simulink library "mechLibrary"  (R2019a)
settings: Solver=VariableStepAuto  StartTime=0.0  StopTime=10.0  RelTol=1e-3
undefined symbols (not defined in the file): X, Y, Z
libraries: sm_lib x45, fl_lib x16, nesl_utility x14, $bdroot x8, servoLibrary x6
(part 1 of 2)
Description:
  | Copyright 2008-2019 The MathWorks, Inc.
  | 
  | Mechanical library
settings Model: Creator=falderis  LastModifiedBy=falderis
settings DataIOCC: ReturnWorkspaceOutputs=off
settings DebuggingCC: ArithmeticOperatorsInVariantConditions=warning

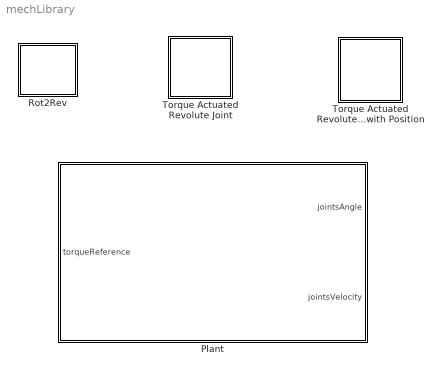
== system mechLibrary ==
  Plant : Subsystem  Description=|
      | Copyright 2008-2019 The MathWorks, Inc.
      | 
      | Mechanical library
      mask Display: image('plant.png')
  Rot2Rev : Subsystem
  Torque Actuated Revolute Joint : Subsystem  mask(Torque actuated revolute joint){angle=0}
      mask prompts: angle "State target for revolute joint (deg)"
      mask Display: image('rev.png');
  Torque Actuated Revolute Joint with Position : Subsystem  mask(Torque actuated revolute joint){angle=0}
      mask prompts: angle "State target for revolute joint (deg)"
      mask Display: image('rev.png');

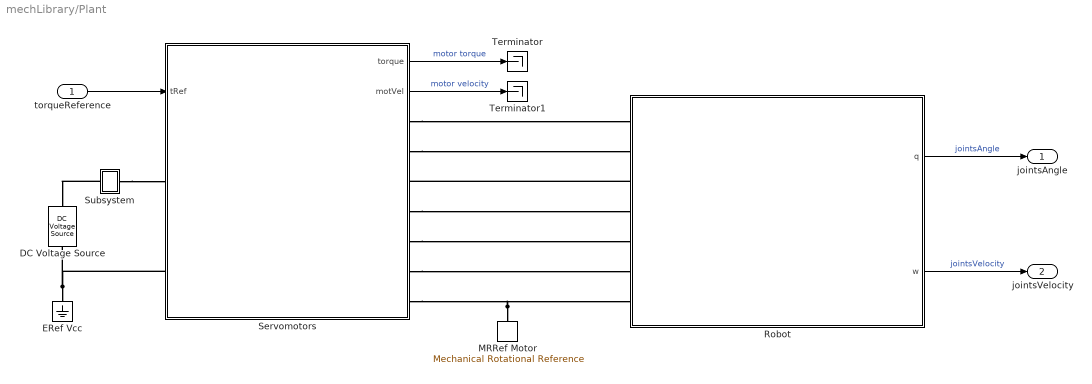
== system mechLibrary/Plant ==
  torqueReference : Inport  OutDataTypeStr=Bus: jointTorqueBus  Unit=N*m
  DC Voltage Source : fl_lib/Electrical/Electrical Sources/DC Voltage Source  v0=12 V
  ERef Vcc : fl_lib/Electrical/Electrical Elements/Electrical Reference
      settings: SourceProductName=Foundation Library
  MRRef Motor : fl_lib/Mechanical/Rotational Elements/Mechanical Rotational Reference
      settings: SourceProductName=Foundation Library
  Robot : Subsystem
      mask Display: image(imread(fullfile(matlabroot,'toolbox','physmod','sm','smdemos','import','robot_stepfiles','images','sm_srobot.png')))
  Servomotors : Subsystem  VariantControl=SV
      mask Display: image('servos.jpg')
  Subsystem : Subsystem
      mask Display: disp('i')
  Terminator : Terminator
  Terminator1 : Terminator
  jointsAngle : Outport  OutDataTypeStr=Bus: jointMotionBus  Unit=deg
  jointsVelocity : Outport  Port=2  OutDataTypeStr=Bus: jointVelBus  Unit=deg/s
  wires:
  Robot/2(w) -> jointsVelocity/1  "jointsVelocity"
  Robot/1(q) -> jointsAngle/1  "jointsAngle"
  Servomotors/2(motVel) -> Terminator1/1  "motor velocity"
  torqueReference/1 -> Servomotors/1(tRef)
  Servomotors/1(torque) -> Terminator/1  "motor torque"
  connections:
  Subsystem/LConn1 -- DC Voltage Source/LConn1
  Subsystem/RConn1 -- Servomotors/LConn1
  Servomotors/RConn6 -- Robot/LConn6
  Servomotors/RConn5 -- Robot/LConn5
  Servomotors/RConn4 -- Robot/LConn4
  Robot/LConn3 -- Servomotors/RConn3
  Servomotors/RConn2 -- Robot/LConn2
  Servomotors/RConn1 -- Robot/LConn1
  ERef Vcc/LConn1 -- DC Voltage Source/RConn1 -- Servomotors/LConn2
  MRRef Motor/LConn1 -- Robot/LConn7 -- Servomotors/RConn7

== system mechLibrary/Rot2Rev ==
  Ideal Angular Velocity Source : fl_lib/Mechanical/Mechanical Sources/Ideal Angular Velocity Source
  Ideal Torque Sensor : fl_lib/Mechanical/Mechanical Sensors/Ideal Torque Sensor
  w : PMIOPort  Side=Right
  R : PMIOPort  Port=2  Side=Right
  t : PMIOPort  Port=3  Side=Left
  C : PMIOPort  Port=4  Side=Left
  connections:
  Ideal Torque Sensor/LConn1 -- Ideal Angular Velocity Source/RConn2
  Ideal Torque Sensor/RConn2 -- t/RConn1
  C/RConn1 -- Ideal Torque Sensor/RConn1
  w/RConn1 -- Ideal Angular Velocity Source/RConn1
  Ideal Angular Velocity Source/LConn1 -- R/RConn1

== system mechLibrary/Torque Actuated Revolute Joint ==
  Rot2Rev : $bdroot/Rot2Rev  SystemSampleTime=-1
  Upper Arm Revolute : sm_lib/Joints/Revolute Joint  SenseConstraintForce=off  SenseConstraintForceX=off  SenseConstraintForceY=off  SenseConstraintForceZ=off  SenseConstraintTorque=off  SenseConstraintTorqueX=off  SenseConstraintTorqueY=off  SenseConstraintTorqueZ=off  SenseTotalForce=off  SenseTotalForceX=off  SenseTotalForceY=off  SenseTotalForceZ=off  SenseTotalTorque=off  SenseTotalTorqueX=off  SenseTotalTorqueY=off  SenseTotalTorqueZ=off  CompositeWrenchDir=FollowerOnBase  CompositeWrenchFrame=BaseFrame  EquilibriumPosition=0  EquilibriumPositionUnits=deg  SpringStiffness=0  SpringStiffnessUnits=N*m/deg  DampingCoefficient=0  DampingCoefficientUnits=N*m/(deg/s)  TorqueActuationMode=InputTorque  MotionActuationMode=ComputedMotion  SensePosition=off  SenseVelocity=on  SenseAcceleration=off  SenseTorqueForce=off  SenseLowerLimitTorqueForce=off  SenseUpperLimitTorqueForce=off  LowerLimitSpecify=off  LowerLimitBound=-90  LowerLimitBoundUnits=deg  LowerLimitStiffness=1e4  LowerLimitStiffnessUnits=N*m/deg  LowerLimitDamping=10  LowerLimitDampingUnits=N*m/(deg/s)  LowerLimitTransitionRegionWidth=0.1  LowerLimitTransitionRegionWidthUnits=deg  UpperLimitSpecify=off  UpperLimitBound=90  UpperLimitBoundUnits=deg  UpperLimitStiffness=1e4  UpperLimitStiffnessUnits=N*m/deg  UpperLimitDamping=10  UpperLimitDampingUnits=N*m/(deg/s)  UpperLimitTransitionRegionWidth=0.1  UpperLimitTransitionRegionWidthUnits=deg  PositionTargetSpecify=on  PositionTargetPriority=Low  PositionTargetValue=angle  PositionTargetValueUnits=deg  VelocityTargetSpecify=off  VelocityTargetPriority=High  VelocityTargetValue=0  VelocityTargetValueUnits=deg/s
  F : PMIOPort  Side=Right
  B : PMIOPort  Port=2  Side=Left
  C : PMIOPort  Port=3  Side=Left
  w : PMIOPort  Port=4  Side=Right
  R : PMIOPort  Port=5  Side=Right
  connections:
  Upper Arm Revolute/RConn2 -- w/RConn1 -- Rot2Rev/RConn1
  Rot2Rev/RConn2 -- R/RConn1
  F/RConn1 -- Upper Arm Revolute/RConn1
  Rot2Rev/LConn1 -- Upper Arm Revolute/LConn2
  B/RConn1 -- Upper Arm Revolute/LConn1
  Rot2Rev/LConn2 -- C/RConn1

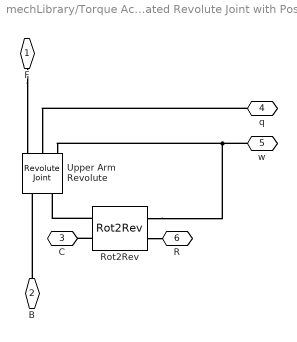
== system mechLibrary/Torque Actuated Revolute Joint with Position ==
  Rot2Rev : $bdroot/Rot2Rev  SystemSampleTime=-1
  Upper Arm Revolute : sm_lib/Joints/Revolute Joint  SenseConstraintForce=off  SenseConstraintForceX=off  SenseConstraintForceY=off  SenseConstraintForceZ=off  SenseConstraintTorque=off  SenseConstraintTorqueX=off  SenseConstraintTorqueY=off  SenseConstraintTorqueZ=off  SenseTotalForce=off  SenseTotalForceX=off  SenseTotalForceY=off  SenseTotalForceZ=off  SenseTotalTorque=off  SenseTotalTorqueX=off  SenseTotalTorqueY=off  SenseTotalTorqueZ=off  CompositeWrenchDir=FollowerOnBase  CompositeWrenchFrame=BaseFrame  EquilibriumPosition=0  EquilibriumPositionUnits=deg  SpringStiffness=0  SpringStiffnessUnits=N*m/deg  DampingCoefficient=0  DampingCoefficientUnits=N*m/(deg/s)  TorqueActuationMode=InputTorque  MotionActuationMode=ComputedMotion  SensePosition=on  SenseVelocity=on  SenseAcceleration=off  SenseTorqueForce=off  SenseLowerLimitTorqueForce=off  SenseUpperLimitTorqueForce=off  LowerLimitSpecify=off  LowerLimitBound=-90  LowerLimitBoundUnits=deg  LowerLimitStiffness=1e4  LowerLimitStiffnessUnits=N*m/deg  LowerLimitDamping=10  LowerLimitDampingUnits=N*m/(deg/s)  LowerLimitTransitionRegionWidth=0.1  LowerLimitTransitionRegionWidthUnits=deg  UpperLimitSpecify=off  UpperLimitBound=90  UpperLimitBoundUnits=deg  UpperLimitStiffness=1e4  UpperLimitStiffnessUnits=N*m/deg  UpperLimitDamping=10  UpperLimitDampingUnits=N*m/(deg/s)  UpperLimitTransitionRegionWidth=0.1  UpperLimitTransitionRegionWidthUnits=deg  PositionTargetSpecify=on  PositionTargetPriority=Low  PositionTargetValue=angle  PositionTargetValueUnits=deg  VelocityTargetSpecify=off  VelocityTargetPriority=High  VelocityTargetValue=0  VelocityTargetValueUnits=deg/s
  F : PMIOPort  Side=Right
  B : PMIOPort  Port=2  Side=Left
  C : PMIOPort  Port=3  Side=Left
  q : PMIOPort  Port=4  Side=Right
  w : PMIOPort  Port=5  Side=Right
  R : PMIOPort  Port=6  Side=Right
  connections:
  Rot2Rev/RConn2 -- R/RConn1
  F/RConn1 -- Upper Arm Revolute/RConn1
  Rot2Rev/LConn1 -- Upper Arm Revolute/LConn2
  B/RConn1 -- Upper Arm Revolute/LConn1
  Rot2Rev/LConn2 -- C/RConn1
  q/RConn1 -- Upper Arm Revolute/RConn2
  w/RConn1 -- Rot2Rev/RConn1 -- Upper Arm Revolute/RConn3

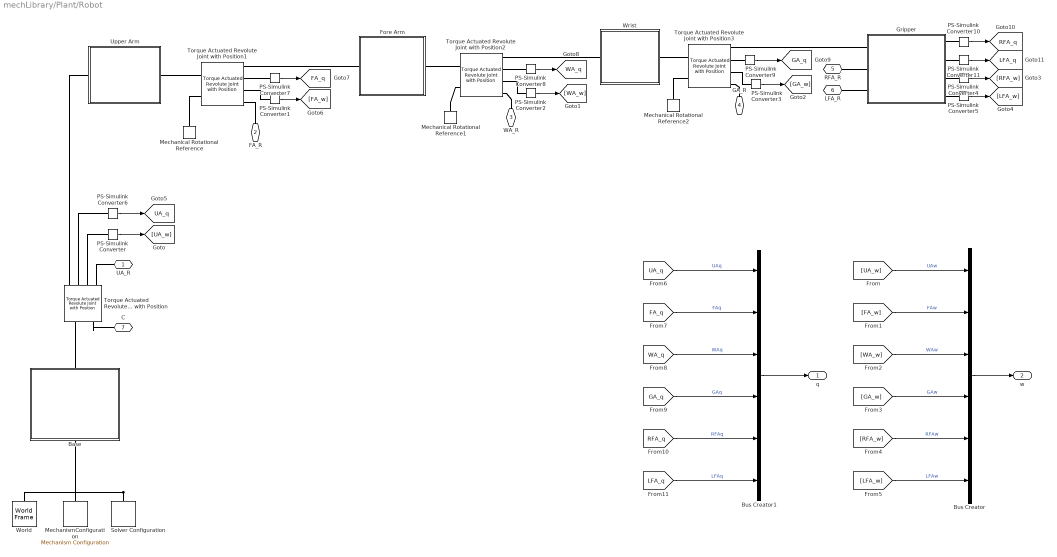
== system mechLibrary/Plant/Robot ==
  Base : Subsystem
      mask Display:
      | image(imread(fullfile(matlabroot,'toolbox','physmod','sm','smdemos','import','robot_stepfiles','images','sm_srobot_base.png')));
      | port_label('LConn',1,'B')
      | port_label('RConn',1,'F')
  Bus Creator : BusCreator  Inputs=6  OutDataTypeStr=Bus: jointVelBus
      settings: InheritFromInputs=off
  Bus Creator1 : BusCreator  Inputs=6  OutDataTypeStr=Bus: jointMotionBus
      settings: InheritFromInputs=off
  Fore Arm : Subsystem
      mask Display:
      | image(imread(fullfile(matlabroot,'toolbox','physmod','sm','smdemos','import','robot_stepfiles','images','sm_srobot_forearm.png')))
      | port_label('LConn',1,'B')
      | port_label('RConn',1,'F')
  Gripper : Subsystem
      mask Display:
      | image(imread(fullfile(matlabroot,'toolbox','physmod','sm','smdemos','import','robot_stepfiles','images','sm_srobot_grip.png')))
      | port_label('LConn',1,'Base')
  Mechanical Rotational Reference : fl_lib/Mechanical/Rotational Elements/Mechanical Rotational Reference
  Mechanical Rotational Reference1 : fl_lib/Mechanical/Rotational Elements/Mechanical Rotational Reference
  Mechanical Rotational Reference2 : fl_lib/Mechanical/Rotational Elements/Mechanical Rotational Reference
  MechanismConfiguration : sm_lib/Utilities/Mechanism Configuration  UniformGravity=Constant  GravityVector=[0 -9.81 0]  GravityUnits=m/s^2  LinearizationDelta=0.001
  PS-Simulink Converter{,1..5} (6 alike) : nesl_utility/PS-Simulink Converter  PhysicalDomain=network_engine_domain  SubClassName=ps_output  LeftPortType=input  RightPortType=output  PseudoPeriodic=off  Frequencies=[]  Unit=deg/s  AffineConversion=off
  PS-Simulink Converter{6..11} (6 alike) : nesl_utility/PS-Simulink Converter  PhysicalDomain=network_engine_domain  SubClassName=ps_output  LeftPortType=input  RightPortType=output  PseudoPeriodic=off  Frequencies=[]  Unit=deg  AffineConversion=off
  Solver Configuration : nesl_utility/Solver Configuration  PhysicalDomain=network_engine_domain  SubClassName=solver  LeftPortType=input  RightPortType=generic  Tones=[]  Harmonics=[]  SimulateNoise=off  Profile=off  UseLocalSampling=off  EnableSwitchedLinearOptims=on  FrequencyDomain=off  UseCCode=off  RelTol=0.001  AbsTol=1e-06  MinStep=1e-09  ToWorkspace=off  RevertToSquareIcSolve=off  NumHomotopyIterations=100  PhasorMode=off  PhasorModeNumHarmonics=1  DoDC=off  ResidualTolerance=1e-09  UseLocalSolver=off  LocalSolverChoice=NE_BACKWARD_EULER_ADVANCER  LocalSolverSampleTime=0.001  DoFixedCost=off  MaxNonlinIter=3  MaxModeIter=2  LinearAlgebra=Sparse  EquationFormulation=NE_TIME_EF  DelaysMemoryBudget=1024  AutomaticFiltering=on  FilteringTimeConstant=0.001  PartitionStorageMethod=AS_NEEDED  PartitionMemoryBudget=1024  PartitionMethod=FAST
  Torque Actuated Revolute Joint with Position{,1..3} (4 alike) : $bdroot/Torque Actuated Revolute Joint with Position  angle=0
  Upper Arm : Subsystem
      mask Display:
      | image(imread(fullfile(matlabroot,'toolbox','physmod','sm','smdemos','import','robot_stepfiles','images','sm_srobot_upperarm.png')))
      | port_label('LConn',1,'B')
      | port_label('RConn',1,'F')
  World : sm_lib/Frames and Transforms/World Frame
  Wrist : Subsystem
      mask Display:
      | image(imread(fullfile(matlabroot,'toolbox','physmod','sm','smdemos','import','robot_stepfiles','images','sm_srobot_wrist.png')))
      | port_label('LConn',1,'B')
      | port_label('RConn',1,'F')
  UA_R : PMIOPort  Side=Left
  FA_R : PMIOPort  Port=2  Side=Left
  WA_R : PMIOPort  Port=3  Side=Left
  GA_R : PMIOPort  Port=4  Side=Left
  RFA_R : PMIOPort  Port=5  Side=Left
  LFA_R : PMIOPort  Port=6  Side=Left
  C : PMIOPort  Port=7  Side=Left
  q : Outport  OutDataTypeStr=Bus: jointMotionBus  Unit=deg
  w : Outport  Port=2  OutDataTypeStr=Bus: jointVelBus  Unit=deg/s
  tag scope: FA_q=global, GA_q=global, LFA_q=global, RFA_q=global, UA_q=global, WA_q=global
  wires:
  [LFA_q] -> Bus Creator1/6  "LFAq"
  [RFA_q] -> Bus Creator1/5  "RFAq"
  [GA_q] -> Bus Creator1/4  "GAq"
  [WA_q] -> Bus Creator1/3  "WAq"
  [FA_q] -> Bus Creator1/2  "FAq"
  [UA_q] -> Bus Creator1/1  "UAq"
  PS-Simulink Converter9/1 -> [GA_q]
  PS-Simulink Converter3/1 -> [GA_w]
  PS-Simulink Converter1/1 -> [FA_w]
  PS-Simulink Converter2/1 -> [WA_w]
  PS-Simulink Converter/1 -> [UA_w]
  PS-Simulink Converter4/1 -> [RFA_w]
  PS-Simulink Converter6/1 -> [UA_q]
  PS-Simulink Converter8/1 -> [WA_q]
  PS-Simulink Converter7/1 -> [FA_q]
  PS-Simulink Converter5/1 -> [LFA_w]
  PS-Simulink Converter10/1 -> [RFA_q]
  PS-Simulink Converter11/1 -> [LFA_q]
  Bus Creator1/1 -> q/1
  [LFA_w] -> Bus Creator/6  "LFAw"
  [RFA_w] -> Bus Creator/5  "RFAw"
  [GA_w] -> Bus Creator/4  "GAw"
  [WA_w] -> Bus Creator/3  "WAw"
  Bus Creator/1 -> w/1
  [FA_w] -> Bus Creator/2  "FAw"
  [UA_w] -> Bus Creator/1  "UAw"
  connections:
  PS-Simulink Converter8/LConn1 -- Torque Actuated Revolute Joint with Position2/RConn2
  Mechanical Rotational Reference1/LConn1 -- Torque Actuated Revolute Joint with Position2/LConn2
  Torque Actuated Revolute Joint with Position/RConn4 -- UA_R/RConn1
  Torque Actuated Revolute Joint with Position3/RConn3 -- PS-Simulink Converter3/LConn1
  Torque Actuated Revolute Joint with Position1/LConn2 -- Mechanical Rotational Reference/LConn1
  Torque Actuated Revolute Joint with Position3/RConn1 -- Gripper/LConn1
  GA_R/RConn1 -- Torque Actuated Revolute Joint with Position3/RConn4
  Gripper/LConn3 -- LFA_R/RConn1
  Torque Actuated Revolute Joint with Position/RConn2 -- PS-Simulink Converter6/LConn1
  PS-Simulink Converter10/LConn1 -- Gripper/RConn1
  Torque Actuated Revolute Joint with Position/LConn2 -- C/RConn1
  PS-Simulink Converter7/LConn1 -- Torque Actuated Revolute Joint with Position1/RConn2
  Torque Actuated Revolute Joint with Position/LConn1 -- Base/RConn1
  Torque Actuated Revolute Joint with Position3/LConn1 -- Wrist/RConn1
  Torque Actuated Revolute Joint with Position2/RConn1 -- Wrist/LConn1
  RFA_R/RConn1 -- Gripper/LConn2
  Torque Actuated Revolute Joint with Position/RConn1 -- Upper Arm/LConn1
  Mechanical Rotational Reference2/LConn1 -- Torque Actuated Revolute Joint with Position3/LConn2
  Fore Arm/LConn1 -- Torque Actuated Revolute Joint with Position1/RConn1
  Gripper/RConn3 -- PS-Simulink Converter4/LConn1
  Torque Actuated Revolute Joint with Position2/RConn3 -- PS-Simulink Converter2/LConn1
  FA_R/RConn1 -- Torque Actuated Revolute Joint with Position1/RConn4
  Torque Actuated Revolute Joint with Position3/RConn2 -- PS-Simulink Converter9/LConn1
  Torque Actuated Revolute Joint with Position1/LConn1 -- Upper Arm/RConn1
  WA_R/RConn1 -- Torque Actuated Revolute Joint with Position2/RConn4
  Gripper/RConn2 -- PS-Simulink Converter11/LConn1
  PS-Simulink Converter/LConn1 -- Torque Actuated Revolute Joint with Position/RConn3
  Torque Actuated Revolute Joint with Position2/LConn1 -- Fore Arm/RConn1
  Gripper/RConn4 -- PS-Simulink Converter5/LConn1
  Torque Actuated Revolute Joint with Position1/RConn3 -- PS-Simulink Converter1/LConn1
  Solver Configuration/RConn1 -- Base/LConn1 -- World/RConn1 -- MechanismConfiguration/RConn1

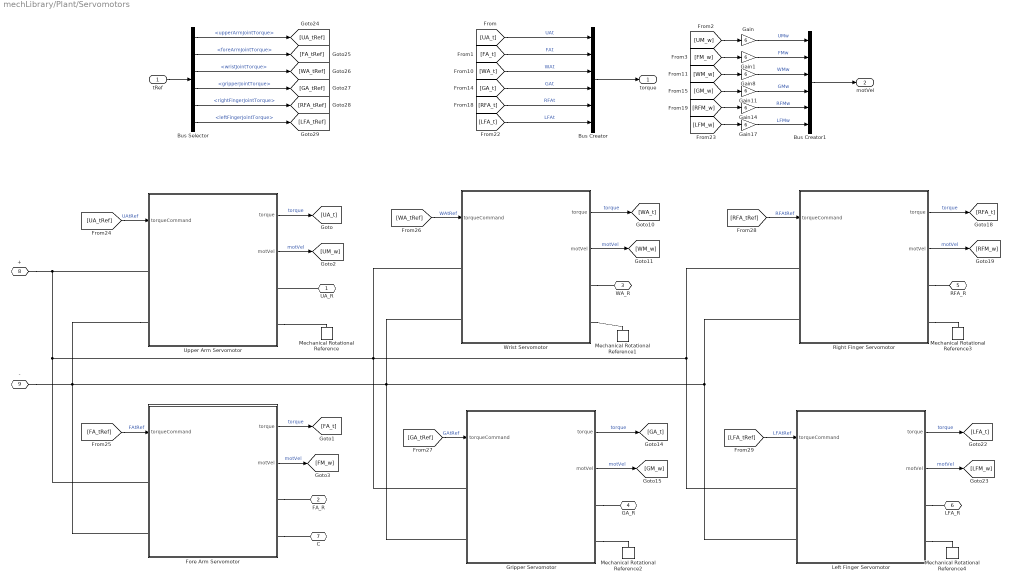
== system mechLibrary/Plant/Servomotors ==
  tRef : Inport  OutDataTypeStr=Bus: jointTorqueBus  Unit=N*m
  Bus Creator : BusCreator  Inputs=6  OutDataTypeStr=Bus: jointTorqueBus
      settings: InheritFromInputs=off
  Bus Creator1 : BusCreator  Inputs=6  OutDataTypeStr=Bus: jointVelBus
      settings: InheritFromInputs=off
  Bus Selector : BusSelector  OutputSignals=upperArmJointTorque,foreArmJointTorque,wristJointTorque,gripperJointTorque,rightFingerJointTorque,leftFingerJointTorque
  Fore Arm Servomotor : Subsystem  Tag=PublishSubsystem  mask(Servomotor){T_iMask=1e-3, etaMask=100, rpm_etaMask=3000, trq_etaMask=0.955, trq_stallMask=4, rpm_maxMask=5000, JMask=0.173*1e-4, rpm0Mask=0, gearRatioMask=10}
      mask prompts: T_iMask "Current loop time constant (s)"; etaMask "Efficiency (%)"; rpm_etaMask "Speed at which efficiency measured (rpm)"; trq_etaMask "Torque at which efficiency measured  (Nm)"; trq_stallMask "Stall torque (Nm)"; rpm_maxMask "Maximum speed (rpm)"; JMask "Rotor inertia (kg*m^2)"; rpm0Mask "Rotor initial speed (rpm)"; gearRatioMask "Gearbox ratio"
      mask help: Implements an abstracted model of a servomotor and driver.
      mask DialogControl ParameterTabVar0 Prompt: Electrical
      mask DialogControl ParameterTabVar01 Prompt: Efficiency
      mask DialogControl ParameterTabVar012 Prompt: Mechanical
      mask Display: image('servo.jpg')
  Gain{,1,8,11,14,17} (6 alike) : Gain  Gain=6
  Gripper Servomotor : Subsystem  Tag=PublishSubsystem  mask(Servomotor){T_iMask=1e-3, etaMask=100, rpm_etaMask=3000, trq_etaMask=0.637, trq_stallMask=1.9, rpm_maxMask=5000, JMask=0.193*1e-4, rpm0Mask=0, gearRatioMask=1}
      mask prompts: T_iMask "Current loop time constant (s)"; etaMask "Efficiency (%)"; rpm_etaMask "Speed at which efficiency measured (rpm)"; trq_etaMask "Torque at which efficiency measured  (Nm)"; trq_stallMask "Stall torque (Nm)"; rpm_maxMask "Maximum speed (rpm)"; JMask "Rotor inertia (kg*m^2)"; rpm0Mask "Rotor initial speed (rpm)"; gearRatioMask "Gearbox ratio"
      mask help: Implements an abstracted model of a servomotor and driver.
      mask DialogControl ParameterTabVar0 Prompt: Electrical
      mask DialogControl ParameterTabVar01 Prompt: Efficiency
      mask DialogControl ParameterTabVar012 Prompt: Mechanical
      mask Display: image('servo.jpg')
  Left Finger Servomotor : Subsystem  Tag=PublishSubsystem  mask(Servomotor){T_iMask=1e-3, etaMask=100, rpm_etaMask=3000, trq_etaMask=0.637, trq_stallMask=1.9, rpm_maxMask=5000, JMask=0.193*1e-4, rpm0Mask=0, gearRatioMask=5}
      mask prompts: T_iMask "Current loop time constant (s)"; etaMask "Efficiency (%)"; rpm_etaMask "Speed at which efficiency measured (rpm)"; trq_etaMask "Torque at which efficiency measured  (Nm)"; trq_stallMask "Stall torque (Nm)"; rpm_maxMask "Maximum speed (rpm)"; JMask "Rotor inertia (kg*m^2)"; rpm0Mask "Rotor initial speed (rpm)"; gearRatioMask "Gearbox ratio"
      mask help: Implements an abstracted model of a servomotor and driver.
      mask DialogControl ParameterTabVar0 Prompt: Electrical
      mask DialogControl ParameterTabVar01 Prompt: Efficiency
      mask DialogControl ParameterTabVar012 Prompt: Mechanical
      mask Display: image('servo.jpg')
  Mechanical Rotational Reference{,1..4} (5 alike) : fl_lib/Mechanical/Rotational Elements/Mechanical Rotational Reference
  Right Finger Servomotor : Subsystem  Tag=PublishSubsystem  mask(Servomotor){T_iMask=1e-3, etaMask=100, rpm_etaMask=3000, trq_etaMask=0.637, trq_stallMask=1.9, rpm_maxMask=5000, JMask=0.193*1e-4, rpm0Mask=0, gearRatioMask=5}
      mask prompts: T_iMask "Current loop time constant (s)"; etaMask "Efficiency (%)"; rpm_etaMask "Speed at which efficiency measured (rpm)"; trq_etaMask "Torque at which efficiency measured  (Nm)"; trq_stallMask "Stall torque (Nm)"; rpm_maxMask "Maximum speed (rpm)"; JMask "Rotor inertia (kg*m^2)"; rpm0Mask "Rotor initial speed (rpm)"; gearRatioMask "Gearbox ratio"
      mask help: Implements an abstracted model of a servomotor and driver.
      mask DialogControl ParameterTabVar0 Prompt: Electrical
      mask DialogControl ParameterTabVar01 Prompt: Efficiency
      mask DialogControl ParameterTabVar012 Prompt: Mechanical
      mask Display: image('servo.jpg')
  Upper Arm Servomotor : Subsystem  Tag=PublishSubsystem  VariantControl=SV  mask(Servomotor){T_iMask=1e-3, etaMask=100, rpm_etaMask=3000, trq_etaMask=2.07, trq_stallMask=7, rpm_maxMask=5000, JMask=0.672*1e-4, rpm0Mask=0, gearRatioMask=10}
      mask prompts: T_iMask "Current loop time constant (s)"; etaMask "Efficiency (%)"; rpm_etaMask "Speed at which efficiency measured (rpm)"; trq_etaMask "Torque at which efficiency measured  (Nm)"; trq_stallMask "Stall torque (Nm)"; rpm_maxMask "Maximum speed (rpm)"; JMask "Rotor inertia (kg*m^2)"; rpm0Mask "Rotor initial speed (rpm)"; gearRatioMask "Gearbox ratio"
      mask help: Implements an abstracted model of a servomotor and driver.
      mask DialogControl ParameterTabVar0 Prompt: Electrical
      mask DialogControl ParameterTabVar01 Prompt: Efficiency
      mask DialogControl ParameterTabVar012 Prompt: Mechanical
      mask Display: image('servo.jpg')
  Wrist Servomotor : Subsystem  Tag=PublishSubsystem  mask(Servomotor){T_iMask=1e-3, etaMask=100, rpm_etaMask=3000, trq_etaMask=0.955, trq_stallMask=4, rpm_maxMask=5000, JMask=0.173*1e-4, rpm0Mask=0, gearRatioMask=50}
      mask prompts: T_iMask "Current loop time constant (s)"; etaMask "Efficiency (%)"; rpm_etaMask "Speed at which efficiency measured (rpm)"; trq_etaMask "Torque at which efficiency measured  (Nm)"; trq_stallMask "Stall torque (Nm)"; rpm_maxMask "Maximum speed (rpm)"; JMask "Rotor inertia (kg*m^2)"; rpm0Mask "Rotor initial speed (rpm)"; gearRatioMask "Gearbox ratio"
      mask help: Implements an abstracted model of a servomotor and driver.
      mask DialogControl ParameterTabVar0 Prompt: Electrical
      mask DialogControl ParameterTabVar01 Prompt: Efficiency
      mask DialogControl ParameterTabVar012 Prompt: Mechanical
      mask Display: image('servo.jpg')
  UA_R : PMIOPort  Side=Right
  FA_R : PMIOPort  Port=2  Side=Right
  WA_R : PMIOPort  Port=3  Side=Right
  GA_R : PMIOPort  Port=4  Side=Right
  RFA_R : PMIOPort  Port=5  Side=Right
  LFA_R : PMIOPort  Port=6  Side=Right
  C : PMIOPort  Port=7  Side=Right
  + : PMIOPort  Port=8  Side=Left
  - : PMIOPort  Port=9  Side=Left
  torque : Outport  OutDataTypeStr=Bus: jointTorqueBus  Unit=N*m
  motVel : Outport  Port=2  OutDataTypeStr=Bus: jointVelBus  Unit=deg/s
  wires:
  [UA_tRef] -> Upper Arm Servomotor/1(torqueCommand)  "UAtRef"
  [LFA_tRef] -> Left Finger Servomotor/1(torqueCommand)  "LFAtRef"
  [RFA_tRef] -> Right Finger Servomotor/1(torqueCommand)  "RFAtRef"
  [GA_tRef] -> Gripper Servomotor/1(torqueCommand)  "GAtRef"
  [WA_tRef] -> Wrist Servomotor/1(torqueCommand)  "WAtRef"
  [FA_tRef] -> Fore Arm Servomotor/1(torqueCommand)  "FAtRef"
  Bus Selector/6 -> [LFA_tRef]  "<leftFingerJointTorque>"
  Bus Selector/5 -> [RFA_tRef]  "<rightFingerJointTorque>"
  Bus Selector/4 -> [GA_tRef]  "<gripperJointTorque>"
  Bus Selector/3 -> [WA_tRef]  "<wristJointTorque>"
  Bus Selector/2 -> [FA_tRef]  "<foreArmJointTorque>"
  Bus Selector/1 -> [UA_tRef]  "<upperArmJointTorque>"
  tRef/1 -> Bus Selector/1
  [LFM_w] -> Gain17/1
  Gain17/1 -> Bus Creator1/6  "LFMw"
  Left Finger Servomotor/2(motVel) -> [LFM_w]  "motVel"
  Left Finger Servomotor/1(torque) -> [LFA_t]  "torque"
  Gain14/1 -> Bus Creator1/5  "RFMw"
  [RFM_w] -> Gain14/1
  Right Finger Servomotor/2(motVel) -> [RFM_w]  "motVel"
  Right Finger Servomotor/1(torque) -> [RFA_t]  "torque"
  Gain11/1 -> Bus Creator1/4  "GMw"
  [GM_w] -> Gain11/1
  Gripper Servomotor/1(torque) -> [GA_t]  "torque"
  Gripper Servomotor/2(motVel) -> [GM_w]  "motVel"
  Gain8/1 -> Bus Creator1/3  "WMw"
  [WM_w] -> Gain8/1
  Wrist Servomotor/1(torque) -> [WA_t]  "torque"
  Wrist Servomotor/2(motVel) -> [WM_w]  "motVel"
  [LFA_t] -> Bus Creator/6  "LFAt"
  [RFA_t] -> Bus Creator/5  "RFAt"
  [GA_t] -> Bus Creator/4  "GAt"
  [WA_t] -> Bus Creator/3  "WAt"
  [FA_t] -> Bus Creator/2  "FAt"
  [UA_t] -> Bus Creator/1  "UAt"
  Gain1/1 -> Bus Creator1/2  "FMw"
  [FM_w] -> Gain1/1
  Gain/1 -> Bus Creator1/1  "UMw"
  [UM_w] -> Gain/1
  Bus Creator1/1 -> motVel/1
  Fore Arm Servomotor/2(motVel) -> [FM_w]  "motVel"
  Upper Arm Servomotor/2(motVel) -> [UM_w]  "motVel"
  Bus Creator/1 -> torque/1
  Fore Arm Servomotor/1(torque) -> [FA_t]  "torque"
  Upper Arm Servomotor/1(torque) -> [UA_t]  "torque"
  connections:
  Upper Arm Servomotor/LConn2 -- Gripper Servomotor/LConn2 -- Left Finger Servomotor/LConn2 -- Right Finger Servomotor/LConn2 -- Wrist Servomotor/LConn2 -- Fore Arm Servomotor/LConn2 -- -/RConn1
  +/RConn1 -- Wrist Servomotor/LConn1 -- Gripper Servomotor/LConn1 -- Right Finger Servomotor/LConn1 -- Left Finger Servomotor/LConn1 -- Fore Arm Servomotor/LConn1 -- Upper Arm Servomotor/LConn1
  Left Finger Servomotor/RConn1 -- LFA_R/RConn1
  Left Finger Servomotor/RConn2 -- Mechanical Rotational Reference4/LConn1
  Right Finger Servomotor/RConn1 -- RFA_R/RConn1
  Right Finger Servomotor/RConn2 -- Mechanical Rotational Reference3/LConn1
  Gripper Servomotor/RConn1 -- GA_R/RConn1
  Gripper Servomotor/RConn2 -- Mechanical Rotational Reference2/LConn1
  Wrist Servomotor/RConn1 -- WA_R/RConn1
  Wrist Servomotor/RConn2 -- Mechanical Rotational Reference1/LConn1
  Fore Arm Servomotor/RConn1 -- FA_R/RConn1
  UA_R/RConn1 -- Upper Arm Servomotor/RConn1
  Upper Arm Servomotor/RConn2 -- Mechanical Rotational Reference/LConn1
  Fore Arm Servomotor/RConn2 -- C/RConn1

== system mechLibrary/Plant/Subsystem ==
  Current Sensor : fl_lib/Electrical/Electrical Sensors/Current Sensor
  PS-Simulink Converter : nesl_utility/PS-Simulink Converter  PhysicalDomain=network_engine_domain  SubClassName=ps_output  LeftPortType=input  RightPortType=output  PseudoPeriodic=off  Frequencies=[]  Unit=A  AffineConversion=off
  Terminator : Terminator
  - : PMIOPort  Side=Right
  + : PMIOPort  Port=2  Side=Left
  wires:
  PS-Simulink Converter/1 -> Terminator/1  "i"
  connections:
  Current Sensor/RConn2 -- -/RConn1
  Current Sensor/LConn1 -- +/RConn1
  PS-Simulink Converter/LConn1 -- Current Sensor/RConn1

== system mechLibrary/Plant/Robot/Base ==
  Follower Transform : sm_lib/Frames and Transforms/Rigid Transform  TranslationMethod=Cartesian  TranslationStandardOffset=0  TranslationLengthUnit=cm  TranslationStandardAxis=+Z  TranslationCartesianOffset=[-1.27 13.219501833114727 0]  TranslationROffset=0  TranslationROffsetUnits=m  TranslationZOffset=0  TranslationZOffsetUnits=m  TranslationThetaOffset=0  TranslationThetaOffsetUnits=deg  RotationMethod=AlignedAxes  RotationAngleUnits=rad  RotationStandardAxis=+X  RotationAngle=0  RotationArbitraryAxis=[0 0 0]  FollAlignAxisA=+Z  BaseAlignAxisA=+Y  FollAlignAxisB=+Y  BaseAlignAxisB=-Z  RotationSequenceAxes=FollowerAxes  RotationSequence=XYX  RotationSequenceAngles=[0 0 0]  RotationSequenceAnglesUnits=deg  RotationMatrix=[1 0 0; 0 1 0; 0 0 1]
  Solid : sm_lib/Body Elements/Solid  InertiaType=CalculateFromGeometry  Mass=9.4647342056355477  MassUnits=kg  CenterOfMass=[-2.8401280055298526 2.356457036499791 1.9022671409295064e-06]  CenterOfMassUnits=cm  MomentsOfInertia=[198.05155722256725 401.13319070315077 274.27880092722387]  MomentsOfInertiaUnits=kg*cm^2  ProductsOfInertia=[-4.2350153206174201e-05 -5.3173128870773767e-05 -2.7282029843043611]  ProductsOfInertiaUnits=kg*cm^2  BasedOnType=Mass  Density=1000  DensityUnits=kg/(m^3)  DoExposeReferenceFrame=on  SerializedFrames=<Frames/>  GraphicType=FromGeometry  MarkerShape=Sphere  MarkerSize=10  MarkerSizeUnits=m  GraphicVisPropType=SimpleVisualProperties  GraphicDiffuseColor=[0.6470588235294118 0.81960784313725488 0.81960784313725488]  GraphicSpecularColor=[0.5 0.5 0.5 1.0]  GraphicAmbientColor=[0.15 0.15 0.15 1.0]  GraphicEmissiveColor=[0.0 0.0 0.0 1.0]  GraphicShininess=75  GraphicOpacity=1  GeometryShape=FromFile  RectangleSize=[1 1]  RectangleSizeUnits=m  BrickDimensions=[1 1 1]  BrickDimensionUnits=m  CylinderRadius=1  CylinderRadiusUnits=m  CylinderLength=1  CylinderLengthUnits=m  SphereRadius=1  SphereRadiusUnits=m  EllipsoidRadii=[1 1 1]  EllipsoidRadiiUnits=m  ExtrusionCrossSection=[1 1; -1 1; -1 -1; 1 -1]  ExtrusionCrossSectionUnits=m  ExtrusionLength=1  ExtrusionLengthUnits=m  PolygonNumSides=3  PolygonOuterRadius=1  PolygonOuterRadiusUnits=m  ExtGeomFileType=STEP  ExtGeomFileName=sm_srobot_base.step  ExtGeomFileUnits=cm  RevolutionCrossSection=[1 1; 1 -1; 2 -1; 2 1]  RevolutionCrossSectionUnits=m  RevolutionExtent=Full  RevolutionAngle=180  RevolutionAngleUnits=deg
  B : PMIOPort  Side=Left
  F : PMIOPort  Port=2  Side=Right
  connections:
  Follower Transform/RConn1 -- F/RConn1
  Follower Transform/LConn1 -- B/RConn1 -- Solid/RConn1

== system mechLibrary/Plant/Robot/Fore Arm ==
  Base Transform : sm_lib/Frames and Transforms/Rigid Transform  TranslationMethod=Cartesian  TranslationStandardOffset=0  TranslationLengthUnit=cm  TranslationStandardAxis=+Z  TranslationCartesianOffset=[-1.651 -4.3948194200880408 0]  TranslationROffset=0  TranslationROffsetUnits=m  TranslationZOffset=0  TranslationZOffsetUnits=m  TranslationThetaOffset=0  TranslationThetaOffsetUnits=deg  RotationMethod=ArbitraryAxis  RotationAngleUnits=deg  RotationStandardAxis=+Z  RotationAngle=120  RotationArbitraryAxis=[-1 -1 -1]  FollAlignAxisA=+X  BaseAlignAxisA=+Y  FollAlignAxisB=+Y  BaseAlignAxisB=+Z  RotationSequenceAxes=FollowerAxes  RotationSequence=XYX  RotationSequenceAngles=[0 0 0]  RotationSequenceAnglesUnits=deg  RotationMatrix=[1 0 0; 0 1 0; 0 0 1]
  Follower Transform : sm_lib/Frames and Transforms/Rigid Transform  TranslationMethod=Cartesian  TranslationStandardOffset=0  TranslationLengthUnit=cm  TranslationStandardAxis=+Z  TranslationCartesianOffset=[9.271 0 -4.6234194200880419]  TranslationROffset=0  TranslationROffsetUnits=m  TranslationZOffset=0  TranslationZOffsetUnits=m  TranslationThetaOffset=0  TranslationThetaOffsetUnits=deg  RotationMethod=ArbitraryAxis  RotationAngleUnits=rad  RotationStandardAxis=+Z  RotationAngle=0  RotationArbitraryAxis=[0 0 0]  FollAlignAxisA=+X  BaseAlignAxisA=+Y  FollAlignAxisB=+Y  BaseAlignAxisB=+Z  RotationSequenceAxes=FollowerAxes  RotationSequence=XYX  RotationSequenceAngles=[0 0 0]  RotationSequenceAnglesUnits=deg  RotationMatrix=[1 0 0; 0 1 0; 0 0 1]
  Solid : sm_lib/Body Elements/Solid  InertiaType=CalculateFromGeometry  Mass=1.0045104495138895  MassUnits=kg  CenterOfMass=[4.0422148685586459 0.017780198871457042 -1.6564997076897243e-08]  CenterOfMassUnits=cm  MomentsOfInertia=[2.5694614988167364 11.732862471629781 10.898947046648527]  MomentsOfInertiaUnits=kg*cm^2  ProductsOfInertia=[-7.4650921853495202e-08 -8.6989013436609002e-08 0.0011574597200765333]  ProductsOfInertiaUnits=kg*cm^2  BasedOnType=Mass  Density=1000  DensityUnits=kg/(m^3)  DoExposeReferenceFrame=on  SerializedFrames=<Frames/>  GraphicType=FromGeometry  MarkerShape=Sphere  MarkerSize=10  MarkerSizeUnits=m  GraphicVisPropType=SimpleVisualProperties  GraphicDiffuseColor=[0.61568627450980395 0.61568627450980395 0.80784313725490198]  GraphicSpecularColor=[0.5 0.5 0.5 1.0]  GraphicAmbientColor=[0.15 0.15 0.15 1.0]  GraphicEmissiveColor=[0.0 0.0 0.0 1.0]  GraphicShininess=75  GraphicOpacity=1  GeometryShape=FromFile  RectangleSize=[1 1]  RectangleSizeUnits=m  BrickDimensions=[1 1 1]  BrickDimensionUnits=m  CylinderRadius=1  CylinderRadiusUnits=m  CylinderLength=1  CylinderLengthUnits=m  SphereRadius=1  SphereRadiusUnits=m  EllipsoidRadii=[1 1 1]  EllipsoidRadiiUnits=m  ExtrusionCrossSection=[1 1; -1 1; -1 -1; 1 -1]  ExtrusionCrossSectionUnits=m  ExtrusionLength=1  ExtrusionLengthUnits=m  PolygonNumSides=3  PolygonOuterRadius=1  PolygonOuterRadiusUnits=m  ExtGeomFileType=STEP  ExtGeomFileName=sm_srobot_forearm.step  ExtGeomFileUnits=cm  RevolutionCrossSection=[1 1; 1 -1; 2 -1; 2 1]  RevolutionCrossSectionUnits=m  RevolutionExtent=Full  RevolutionAngle=180  RevolutionAngleUnits=deg
  B : PMIOPort  Side=Left
  F : PMIOPort  Port=2  Side=Right
  connections:
  Base Transform/RConn1 -- B/RConn1
  Follower Transform/RConn1 -- F/RConn1
  Base Transform/LConn1 -- Follower Transform/LConn1 -- Solid/RConn1

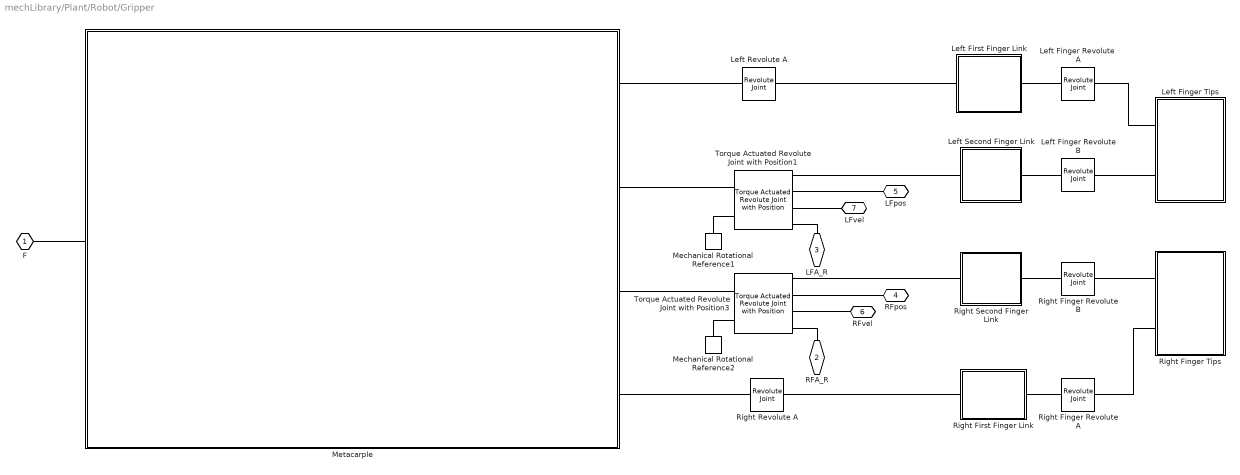
== system mechLibrary/Plant/Robot/Gripper ==
  Left Finger Revolute  A : sm_lib/Joints/Revolute Joint  SenseConstraintForce=off  SenseConstraintForceX=off  SenseConstraintForceY=off  SenseConstraintForceZ=off  SenseConstraintTorque=off  SenseConstraintTorqueX=off  SenseConstraintTorqueY=off  SenseConstraintTorqueZ=off  SenseTotalForce=off  SenseTotalForceX=off  SenseTotalForceY=off  SenseTotalForceZ=off  SenseTotalTorque=off  SenseTotalTorqueX=off  SenseTotalTorqueY=off  SenseTotalTorqueZ=off  CompositeWrenchDir=FollowerOnBase  CompositeWrenchFrame=BaseFrame  EquilibriumPosition=0  EquilibriumPositionUnits=rad  SpringStiffness=0  SpringStiffnessUnits=m*N/rad  DampingCoefficient=0  DampingCoefficientUnits=m*s*N/rad  TorqueActuationMode=NoTorque  MotionActuationMode=ComputedMotion  SensePosition=off  SenseVelocity=off  SenseAcceleration=off  SenseTorqueForce=off  SenseLowerLimitTorqueForce=off  SenseUpperLimitTorqueForce=off  LowerLimitSpecify=off  LowerLimitBound=-90  LowerLimitBoundUnits=deg  LowerLimitStiffness=1e4  LowerLimitStiffnessUnits=N*m/deg  LowerLimitDamping=10  LowerLimitDampingUnits=N*m/(deg/s)  LowerLimitTransitionRegionWidth=0.1  LowerLimitTransitionRegionWidthUnits=deg  UpperLimitSpecify=off  UpperLimitBound=90  UpperLimitBoundUnits=deg  UpperLimitStiffness=1e4  UpperLimitStiffnessUnits=N*m/deg  UpperLimitDamping=10  UpperLimitDampingUnits=N*m/(deg/s)  UpperLimitTransitionRegionWidth=0.1  UpperLimitTransitionRegionWidthUnits=deg  PositionTargetSpecify=off  PositionTargetPriority=Low  PositionTargetValue=154.94823075578159  PositionTargetValueUnits=deg  VelocityTargetSpecify=off  VelocityTargetPriority=High  VelocityTargetValue=0  VelocityTargetValueUnits=deg/s
  Left Finger Revolute B : sm_lib/Joints/Revolute Joint  SenseConstraintForce=off  SenseConstraintForceX=off  SenseConstraintForceY=off  SenseConstraintForceZ=off  SenseConstraintTorque=off  SenseConstraintTorqueX=off  SenseConstraintTorqueY=off  SenseConstraintTorqueZ=off  SenseTotalForce=off  SenseTotalForceX=off  SenseTotalForceY=off  SenseTotalForceZ=off  SenseTotalTorque=off  SenseTotalTorqueX=off  SenseTotalTorqueY=off  SenseTotalTorqueZ=off  CompositeWrenchDir=FollowerOnBase  CompositeWrenchFrame=BaseFrame  EquilibriumPosition=0  EquilibriumPositionUnits=rad  SpringStiffness=0  SpringStiffnessUnits=m*N/rad  DampingCoefficient=0  DampingCoefficientUnits=m*s*N/rad  TorqueActuationMode=NoTorque  MotionActuationMode=ComputedMotion  SensePosition=off  SenseVelocity=off  SenseAcceleration=off  SenseTorqueForce=off  SenseLowerLimitTorqueForce=off  SenseUpperLimitTorqueForce=off  LowerLimitSpecify=off  LowerLimitBound=-90  LowerLimitBoundUnits=deg  LowerLimitStiffness=1e4  LowerLimitStiffnessUnits=N*m/deg  LowerLimitDamping=10  LowerLimitDampingUnits=N*m/(deg/s)  LowerLimitTransitionRegionWidth=0.1  LowerLimitTransitionRegionWidthUnits=deg  UpperLimitSpecify=off  UpperLimitBound=90  UpperLimitBoundUnits=deg  UpperLimitStiffness=1e4  UpperLimitStiffnessUnits=N*m/deg  UpperLimitDamping=10  UpperLimitDampingUnits=N*m/(deg/s)  UpperLimitTransitionRegionWidth=0.1  UpperLimitTransitionRegionWidthUnits=deg  PositionTargetSpecify=off  PositionTargetPriority=High  PositionTargetValue=0  PositionTargetValueUnits=deg  VelocityTargetSpecify=off  VelocityTargetPriority=High  VelocityTargetValue=0  VelocityTargetValueUnits=deg/s
  Left Finger Tips : Subsystem
      mask Display:
      | image(imread(fullfile(matlabroot,'toolbox','physmod','sm','smdemos','import','robot_stepfiles','images','sm_srobot_fingertips.png')))
      | port_label('LConn',1,'First')
      | port_label('LConn',2,'Second')
  Left First Finger Link : Subsystem
      mask Display:
      | image(imread(fullfile(matlabroot,'toolbox','physmod','sm','smdemos','import','robot_stepfiles','images','sm_srobot_firstfingerlink.png')))
      | port_label('LConn',1,'B')
      | port_label('RConn',1,'F')
  Left Revolute A : sm_lib/Joints/Revolute Joint  SenseConstraintForce=off  SenseConstraintForceX=off  SenseConstraintForceY=off  SenseConstraintForceZ=off  SenseConstraintTorque=off  SenseConstraintTorqueX=off  SenseConstraintTorqueY=off  SenseConstraintTorqueZ=off  SenseTotalForce=off  SenseTotalForceX=off  SenseTotalForceY=off  SenseTotalForceZ=off  SenseTotalTorque=off  SenseTotalTorqueX=off  SenseTotalTorqueY=off  SenseTotalTorqueZ=off  CompositeWrenchDir=FollowerOnBase  CompositeWrenchFrame=BaseFrame  EquilibriumPosition=0  EquilibriumPositionUnits=rad  SpringStiffness=0  SpringStiffnessUnits=m*N/rad  DampingCoefficient=0  DampingCoefficientUnits=m*s*N/rad  TorqueActuationMode=NoTorque  MotionActuationMode=ComputedMotion  SensePosition=off  SenseVelocity=off  SenseAcceleration=off  SenseTorqueForce=off  SenseLowerLimitTorqueForce=off  SenseUpperLimitTorqueForce=off  LowerLimitSpecify=off  LowerLimitBound=-90  LowerLimitBoundUnits=deg  LowerLimitStiffness=1e4  LowerLimitStiffnessUnits=N*m/deg  LowerLimitDamping=10  LowerLimitDampingUnits=N*m/(deg/s)  LowerLimitTransitionRegionWidth=0.1  LowerLimitTransitionRegionWidthUnits=deg  UpperLimitSpecify=off  UpperLimitBound=90  UpperLimitBoundUnits=deg  UpperLimitStiffness=1e4  UpperLimitStiffnessUnits=N*m/deg  UpperLimitDamping=10  UpperLimitDampingUnits=N*m/(deg/s)  UpperLimitTransitionRegionWidth=0.1  UpperLimitTransitionRegionWidthUnits=deg  PositionTargetSpecify=on  PositionTargetPriority=Low  PositionTargetValue=30  PositionTargetValueUnits=deg  VelocityTargetSpecify=off  VelocityTargetPriority=High  VelocityTargetValue=0  VelocityTargetValueUnits=deg/s
  Left Second Finger Link : Subsystem
      mask Display:
      | image(imread(fullfile(matlabroot,'toolbox','physmod','sm','smdemos','import','robot_stepfiles','images','sm_srobot_secondfingerlink.png')))
      | port_label('LConn',1,'B')
      | port_label('RConn',1,'F')
  Mechanical Rotational Reference1 : fl_lib/Mechanical/Rotational Elements/Mechanical Rotational Reference
  Mechanical Rotational Reference2 : fl_lib/Mechanical/Rotational Elements/Mechanical Rotational Reference
  Metacarple : Subsystem
      mask Display:
      | image(imread(fullfile(matlabroot,'toolbox','physmod','sm','smdemos','import','robot_stepfiles','images','sm_srobot_metacarples.png')))
      | port_label('RConn',1,'A')
      | port_label('RConn',2,'B')
      | port_label('RConn',3,'C')
      | port_label('RConn',4,'D')
  Right Finger Revolute A : sm_lib/Joints/Revolute Joint  SenseConstraintForce=off  SenseConstraintForceX=off  SenseConstraintForceY=off  SenseConstraintForceZ=off  SenseConstraintTorque=off  SenseConstraintTorqueX=off  SenseConstraintTorqueY=off  SenseConstraintTorqueZ=off  SenseTotalForce=off  SenseTotalForceX=off  SenseTotalForceY=off  SenseTotalForceZ=off  SenseTotalTorque=off  SenseTotalTorqueX=off  SenseTotalTorqueY=off  SenseTotalTorqueZ=off  CompositeWrenchDir=FollowerOnBase  CompositeWrenchFrame=BaseFrame  EquilibriumPosition=0  EquilibriumPositionUnits=rad  SpringStiffness=0  SpringStiffnessUnits=m*N/rad  DampingCoefficient=0  DampingCoefficientUnits=m*s*N/rad  TorqueActuationMode=NoTorque  MotionActuationMode=ComputedMotion  SensePosition=off  SenseVelocity=off  SenseAcceleration=off  SenseTorqueForce=off  SenseLowerLimitTorqueForce=off  SenseUpperLimitTorqueForce=off  LowerLimitSpecify=off  LowerLimitBound=-90  LowerLimitBoundUnits=deg  LowerLimitStiffness=1e4  LowerLimitStiffnessUnits=N*m/deg  LowerLimitDamping=10  LowerLimitDampingUnits=N*m/(deg/s)  LowerLimitTransitionRegionWidth=0.1  LowerLimitTransitionRegionWidthUnits=deg  UpperLimitSpecify=off  UpperLimitBound=90  UpperLimitBoundUnits=deg  UpperLimitStiffness=1e4  UpperLimitStiffnessUnits=N*m/deg  UpperLimitDamping=10  UpperLimitDampingUnits=N*m/(deg/s)  UpperLimitTransitionRegionWidth=0.1  UpperLimitTransitionRegionWidthUnits=deg  PositionTargetSpecify=off  PositionTargetPriority=Low  PositionTargetValue=25.051769244218413  PositionTargetValueUnits=deg  VelocityTargetSpecify=off  VelocityTargetPriority=High  VelocityTargetValue=0  VelocityTargetValueUnits=deg/s
  Right Finger Revolute B : sm_lib/Joints/Revolute Joint  SenseConstraintForce=off  SenseConstraintForceX=off  SenseConstraintForceY=off  SenseConstraintForceZ=off  SenseConstraintTorque=off  SenseConstraintTorqueX=off  SenseConstraintTorqueY=off  SenseConstraintTorqueZ=off  SenseTotalForce=off  SenseTotalForceX=off  SenseTotalForceY=off  SenseTotalForceZ=off  SenseTotalTorque=off  SenseTotalTorqueX=off  SenseTotalTorqueY=off  SenseTotalTorqueZ=off  CompositeWrenchDir=FollowerOnBase  CompositeWrenchFrame=BaseFrame  EquilibriumPosition=0  EquilibriumPositionUnits=rad  SpringStiffness=0  SpringStiffnessUnits=m*N/rad  DampingCoefficient=0  DampingCoefficientUnits=m*s*N/rad  TorqueActuationMode=NoTorque  MotionActuationMode=ComputedMotion  SensePosition=off  SenseVelocity=off  SenseAcceleration=off  SenseTorqueForce=off  SenseLowerLimitTorqueForce=off  SenseUpperLimitTorqueForce=off  LowerLimitSpecify=off  LowerLimitBound=-90  LowerLimitBoundUnits=deg  LowerLimitStiffness=1e4  LowerLimitStiffnessUnits=N*m/deg  LowerLimitDamping=10  LowerLimitDampingUnits=N*m/(deg/s)  LowerLimitTransitionRegionWidth=0.1  LowerLimitTransitionRegionWidthUnits=deg  UpperLimitSpecify=off  UpperLimitBound=90  UpperLimitBoundUnits=deg  UpperLimitStiffness=1e4  UpperLimitStiffnessUnits=N*m/deg  UpperLimitDamping=10  UpperLimitDampingUnits=N*m/(deg/s)  UpperLimitTransitionRegionWidth=0.1  UpperLimitTransitionRegionWidthUnits=deg  PositionTargetSpecify=off  PositionTargetPriority=High  PositionTargetValue=0  PositionTargetValueUnits=deg  VelocityTargetSpecify=off  VelocityTargetPriority=High  VelocityTargetValue=0  VelocityTargetValueUnits=deg/s
  Right Finger Tips : Subsystem
      mask Display:
      | image(imread(fullfile(matlabroot,'toolbox','physmod','sm','smdemos','import','robot_stepfiles','images','sm_srobot_fingertips.png')))
      | port_label('LConn',1,'First')
      | port_label('LConn',2,'Second')
  Right First Finger Link : Subsystem
      mask Display:
      | image(imread(fullfile(matlabroot,'toolbox','physmod','sm','smdemos','import','robot_stepfiles','images','sm_srobot_firstfingerlink.png')))
      | port_label('LConn',1,'B')
      | port_label('RConn',1,'F')
  Right Revolute A : sm_lib/Joints/Revolute Joint  SenseConstraintForce=off  SenseConstraintForceX=off  SenseConstraintForceY=off  SenseConstraintForceZ=off  SenseConstraintTorque=off  SenseConstraintTorqueX=off  SenseConstraintTorqueY=off  SenseConstraintTorqueZ=off  SenseTotalForce=off  SenseTotalForceX=off  SenseTotalForceY=off  SenseTotalForceZ=off  SenseTotalTorque=off  SenseTotalTorqueX=off  SenseTotalTorqueY=off  SenseTotalTorqueZ=off  CompositeWrenchDir=FollowerOnBase  CompositeWrenchFrame=BaseFrame  EquilibriumPosition=0  EquilibriumPositionUnits=rad  SpringStiffness=0  SpringStiffnessUnits=m*N/rad  DampingCoefficient=0  DampingCoefficientUnits=m*s*N/rad  TorqueActuationMode=NoTorque  MotionActuationMode=ComputedMotion  SensePosition=off  SenseVelocity=off  SenseAcceleration=off  SenseTorqueForce=off  SenseLowerLimitTorqueForce=off  SenseUpperLimitTorqueForce=off  LowerLimitSpecify=off  LowerLimitBound=-90  LowerLimitBoundUnits=deg  LowerLimitStiffness=1e4  LowerLimitStiffnessUnits=N*m/deg  LowerLimitDamping=10  LowerLimitDampingUnits=N*m/(deg/s)  LowerLimitTransitionRegionWidth=0.1  LowerLimitTransitionRegionWidthUnits=deg  UpperLimitSpecify=off  UpperLimitBound=90  UpperLimitBoundUnits=deg  UpperLimitStiffness=1e4  UpperLimitStiffnessUnits=N*m/deg  UpperLimitDamping=10  UpperLimitDampingUnits=N*m/(deg/s)  UpperLimitTransitionRegionWidth=0.1  UpperLimitTransitionRegionWidthUnits=deg  PositionTargetSpecify=on  PositionTargetPriority=Low  PositionTargetValue=-30  PositionTargetValueUnits=deg  VelocityTargetSpecify=off  VelocityTargetPriority=High  VelocityTargetValue=0  VelocityTargetValueUnits=deg/s
  Right Second Finger Link : Subsystem
      mask Display:
      | image(imread(fullfile(matlabroot,'toolbox','physmod','sm','smdemos','import','robot_stepfiles','images','sm_srobot_secondfingerlink.png')))
      | port_label('LConn',1,'B')
      | port_label('RConn',1,'F')
  Torque Actuated Revolute Joint with Position1 : $bdroot/Torque Actuated Revolute Joint with Position  angle=-123.57
  Torque Actuated Revolute Joint with Position3 : $bdroot/Torque Actuated Revolute Joint with Position  angle=123.57
  F : PMIOPort  Side=Left
  RFA_R : PMIOPort  Tag=PMCPort  Port=2  Side=Left
  LFA_R : PMIOPort  Tag=PMCPort  Port=3  Side=Left
  RFpos : PMIOPort  Port=4  Side=Right
  LFpos : PMIOPort  Port=5  Side=Right
  RFvel : PMIOPort  Port=6  Side=Right
  LFvel : PMIOPort  Port=7  Side=Right
  connections:
  LFpos/RConn1 -- Torque Actuated Revolute Joint with Position1/RConn2
  LFvel/RConn1 -- Torque Actuated Revolute Joint with Position1/RConn3
  Mechanical Rotational Reference1/LConn1 -- Torque Actuated Revolute Joint with Position1/LConn2
  RFpos/RConn1 -- Torque Actuated Revolute Joint with Position3/RConn2
  Mechanical Rotational Reference2/LConn1 -- Torque Actuated Revolute Joint with Position3/LConn2
  Torque Actuated Revolute Joint with Position1/RConn4 -- LFA_R/RConn1
  Torque Actuated Revolute Joint with Position3/RConn3 -- RFvel/RConn1
  RFA_R/RConn1 -- Torque Actuated Revolute Joint with Position3/RConn4
  Right Second Finger Link/LConn1 -- Torque Actuated Revolute Joint with Position3/RConn1
  Left Finger Revolute B/RConn1 -- Left Finger Tips/LConn2
  Right Finger Revolute A/RConn1 -- Right Finger Tips/LConn2
  Right Finger Revolute A/LConn1 -- Right First Finger Link/RConn1
  Left Revolute A/RConn1 -- Left First Finger Link/LConn1
  Left Revolute A/LConn1 -- Metacarple/RConn1
  Torque Actuated Revolute Joint with Position1/RConn1 -- Left Second Finger Link/LConn1
  Torque Actuated Revolute Joint with Position1/LConn1 -- Metacarple/RConn2
  Torque Actuated Revolute Joint with Position3/LConn1 -- Metacarple/RConn3
  Metacarple/LConn1 -- F/RConn1
  Left Finger Revolute  A/RConn1 -- Left Finger Tips/LConn1
  Left Finger Revolute  A/LConn1 -- Left First Finger Link/RConn1
  Left Finger Revolute B/LConn1 -- Left Second Finger Link/RConn1
  Right Finger Revolute B/RConn1 -- Right Finger Tips/LConn1
  Right Finger Revolute B/LConn1 -- Right Second Finger Link/RConn1
  Right Revolute A/RConn1 -- Right First Finger Link/LConn1
  Right Revolute A/LConn1 -- Metacarple/RConn4

== system mechLibrary/Plant/Robot/Upper Arm ==
  Base Transform : sm_lib/Frames and Transforms/Rigid Transform  TranslationMethod=None  TranslationStandardOffset=0  TranslationLengthUnit=cm  TranslationStandardAxis=+Z  TranslationCartesianOffset=[10.033 -4.4964194200880421 0]  TranslationROffset=0  TranslationROffsetUnits=m  TranslationZOffset=0  TranslationZOffsetUnits=m  TranslationThetaOffset=0  TranslationThetaOffsetUnits=deg  RotationMethod=AlignedAxes  RotationAngleUnits=deg  RotationStandardAxis=+Z  RotationAngle=120  RotationArbitraryAxis=[-1 -1 -1]  FollAlignAxisA=+Z  BaseAlignAxisA=+Y  FollAlignAxisB=+Y  BaseAlignAxisB=-Z  RotationSequenceAxes=FollowerAxes  RotationSequence=XYX  RotationSequenceAngles=[0 0 0]  RotationSequenceAnglesUnits=deg  RotationMatrix=[1 0 0; 0 1 0; 0 0 1]
  Follower Transform : sm_lib/Frames and Transforms/Rigid Transform  TranslationMethod=Cartesian  TranslationStandardOffset=0  TranslationLengthUnit=cm  TranslationStandardAxis=+Z  TranslationCartesianOffset=[10.033 -4.4964194200880421 0]  TranslationROffset=0  TranslationROffsetUnits=m  TranslationZOffset=0  TranslationZOffsetUnits=m  TranslationThetaOffset=0  TranslationThetaOffsetUnits=deg  RotationMethod=ArbitraryAxis  RotationAngleUnits=deg  RotationStandardAxis=+Z  RotationAngle=120  RotationArbitraryAxis=[-1 -1 -1]  FollAlignAxisA=+X  BaseAlignAxisA=+Y  FollAlignAxisB=+Y  BaseAlignAxisB=+Z  RotationSequenceAxes=FollowerAxes  RotationSequence=XYX  RotationSequenceAngles=[0 0 0]  RotationSequenceAnglesUnits=deg  RotationMatrix=[1 0 0; 0 1 0; 0 0 1]
  Solid : sm_lib/Body Elements/Solid  InertiaType=CalculateFromGeometry  Mass=0.80158119961068475  MassUnits=kg  CenterOfMass=[1.0426561159200607 0.10543225189691562 -5.9975184949751705e-06]  CenterOfMassUnits=in  MomentsOfInertia=[1.0145816000804944 3.8395571109521343 3.6540644347626703]  MomentsOfInertiaUnits=kg*in^2  ProductsOfInertia=[-3.8021587235862617e-06 -8.5269450986053901e-06 0.099164347034999878]  ProductsOfInertiaUnits=kg*in^2  BasedOnType=Mass  Density=1000  DensityUnits=kg/(m^3)  DoExposeReferenceFrame=on  SerializedFrames=<Frames/>  GraphicType=FromGeometry  MarkerShape=Sphere  MarkerSize=10  MarkerSizeUnits=m  GraphicVisPropType=SimpleVisualProperties  GraphicDiffuseColor=[1 0.50980392156862742 0.50980392156862742]  GraphicSpecularColor=[0.5 0.5 0.5 1.0]  GraphicAmbientColor=[0.15 0.15 0.15 1.0]  GraphicEmissiveColor=[0.0 0.0 0.0 1.0]  GraphicShininess=75  GraphicOpacity=1  GeometryShape=FromFile  RectangleSize=[1 1]  RectangleSizeUnits=m  BrickDimensions=[1 1 1]  BrickDimensionUnits=m  CylinderRadius=1  CylinderRadiusUnits=m  CylinderLength=1  CylinderLengthUnits=m  SphereRadius=1  SphereRadiusUnits=m  EllipsoidRadii=[1 1 1]  EllipsoidRadiiUnits=m  ExtrusionCrossSection=[1 1; -1 1; -1 -1; 1 -1]  ExtrusionCrossSectionUnits=m  ExtrusionLength=1  ExtrusionLengthUnits=m  PolygonNumSides=3  PolygonOuterRadius=1  PolygonOuterRadiusUnits=m  ExtGeomFileType=STEP  ExtGeomFileName=sm_srobot_upperarm.step  ExtGeomFileUnits=in  RevolutionCrossSection=[1 1; 1 -1; 2 -1; 2 1]  RevolutionCrossSectionUnits=m  RevolutionExtent=Full  RevolutionAngle=180  RevolutionAngleUnits=deg
  B : PMIOPort  Side=Left
  F : PMIOPort  Port=2  Side=Right
  connections:
  Base Transform/RConn1 -- B/RConn1
  Solid/RConn1 -- Base Transform/LConn1 -- Follower Transform/LConn1
  Follower Transform/RConn1 -- F/RConn1
